simulink model "CAR_CONTROL_SYSTEM"  (R2024b)
settings: Solver=FixedStepAuto  StartTime=0.0  StopTime=inf  FixedStep=1e-3  RelTol=1e-3  EnableMultiTasking=on
model workspace (MAT data in the model file):
  SL_ROS_VariableLengthArrays_MaxSizes : object (value not decoded)
undefined symbols (not defined in the file or in its folder): angular, CIRCUIT, CLTF_DAMP, CLTF_FREQ, CLTF_GAIN, CONTROL, CONTROL_INI, DiscIntNeverNeededParam, dspblkCoreblockFVToolHelper, gcbh, INPUT, linear, MCP3201, MD25, MODEL, MODEL_INI, mpcstate, MPU60X0, MPU9250, MSG, NAV_MPC_CONTROL, OUTPUT, SAMPLING_TIME, SYSID_INPUT, VL6180X
libraries: raspberrypiCommlib x153, simulink x85, raspberrypiNetworklib x8, embedlinuxBasiclib x6, ctrlSharedLib x2, ros2lib x2, mpclib x1, vrlib x1, sldrtlib x1
(part 4 of 16)

== system CAR_CONTROL_SYSTEM/HARDWARE/SENSORS/RCRX iBUS ==
  BUS UPDATE : MATLAB Function  Priority=20  TreatAsAtomicUnit=on
  Data Store Read19 : DataStoreRead  DataStoreName=CONTROL  SampleTime=SAMPLING_TIME  IndexOptions=Index vector (dialog)  Indices=1  OutputSizes=1
  Data Store Write1 : DataStoreWrite  DataStoreName=CONTROL  IndexOptions=Index vector (dialog)  Indices=1  OutputSizes=1
  Display3 : Display
  MATLAB Function : MATLAB Function  TreatAsAtomicUnit=on
  Serial Read1 : raspberrypiCommlib/Serial Read  board=Pi 3 Model B  SCIModule_=/dev/ttyS0  Baudrate_=115200  Parity=None  StopBits_=1  HardwareFlowControl=None  ByteOrder=LittleEndian  DataLength=70  DataType=uint8  OutputStatus=on  SampleTime=SAMPLING_TIME  blockPlatform=RaspberryPi
  Terminator : Terminator
  wires:
  MATLAB Function/1(CH_RAW) -> BUS UPDATE/2(CH_RAW)
  BUS UPDATE/1(CONTROL) -> Data Store Write1/1
  Data Store Read19/1 -> BUS UPDATE/1(CONTROL_IN)
  Serial Read1/1 -> MATLAB Function/1(iBUS_DATA), Display3/1
  Serial Read1/2 -> Terminator/1

== system CAR_CONTROL_SYSTEM/HARDWARE/SENSORS/WALL RANGE SENSOR ==
  ANGLE AND DISTANCE COMPUTATION : Subsystem  TreatAsAtomicUnit=on
      settings: MinAlgLoopOccurrences=on
  Data Store Memory : DataStoreMemory  DataStoreName=REAR_DISTANCE  ReadBeforeWriteMsg=warning  WriteAfterWriteMsg=warning  WriteAfterReadMsg=warning  ShowAdditionalParam=off  OutDataTypeStr=double
  Data Store Memory1 : DataStoreMemory  DataStoreName=FRONT_DISTANCE  ReadBeforeWriteMsg=warning  WriteAfterWriteMsg=warning  WriteAfterReadMsg=warning  ShowAdditionalParam=off  OutDataTypeStr=double
  VL6180X_I2C_FRONT : Subsystem  TreatAsAtomicUnit=on
      settings: MinAlgLoopOccurrences=on  RTWSystemCode=Nonreusable function  FunctionWithSeparateData=on
  VL6180X_I2C_REAR : Subsystem  TreatAsAtomicUnit=on
      settings: MinAlgLoopOccurrences=on  RTWSystemCode=Nonreusable function  FunctionWithSeparateData=on

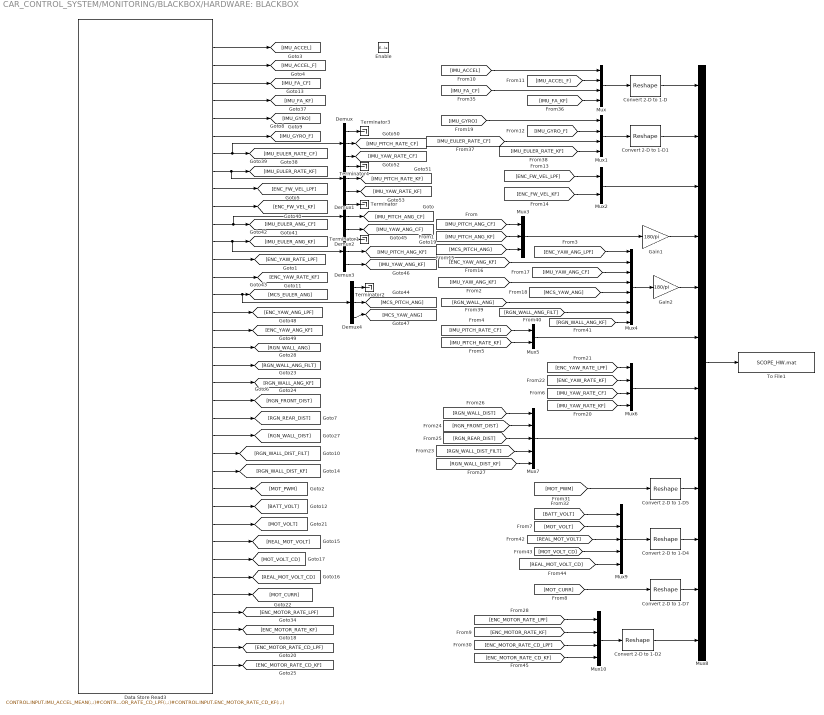
== system CAR_CONTROL_SYSTEM/MONITORING/BLACKBOX/HARDWARE: BLACKBOX ==
  Enable : EnablePort
  Convert 2-D to 1-D{,1..2,4..5,7} (6 alike) : Reshape
  Data Store Read3 : DataStoreRead  DataStoreName=CONTROL  SampleTime=SAMPLING_TIME  DataStoreElements=CONTROL.INPUT.IMU_ACCEL_MEAN(:,:)#CONTROL.INPUT.IMU_ACCEL_MEAN_FILT(:,:)#CONTROL.INPUT.IMU_FORWARD_ACCEL_CF#CONTROL.INPUT.IMU_FORWARD_ACCEL_KF#CONTROL.INPUT.IMU_GYRO_MEAN(:,:)#CONTROL.INPUT.IMU_GYRO_MEAN_FILT(:,:)#CONTROL.INPUT.IMU_EULER_RATE_CF(:,:)#CONTROL.INPUT.IMU_EULER_RATE_KF(:,:)#CONTROL.INPUT.ENC_FORWARD_VEL_LPF#CONTROL.INPUT.ENC_FORWARD_VEL_KF#CONTROL.INPUT.IMU_EULER_ANG_CF(:,:)#CONTROL.INPUT.IMU_EULER_ANG_KF(:,:)#CONTROL.INPUT.ENC_YAW_RATE_LPF#CONTROL.INPUT.ENC_YAW_RATE_KF#CONTROL.INPUT.MCS_EULER_ANG(:,:)#CONTROL.INPUT.ENC_YAW_ANG_LPF#CONTROL.INPUT.ENC_YAW_ANG_KF#CONTROL.INPUT.RANGE_WALL_ANG#CONTROL.INPUT.WALL_ANG_FILT#CONTROL.INPUT.WALL_ANG_KF#CONTROL.INPUT.RANGE_FRONT_DIST#CONTROL.INPUT.RANGE_REAR_DIST#CONTROL.INPUT.RANGE_WALL_DIST#CONTROL.INPUT.WALL_DIST_FILT#CONTROL.INPUT.WALL_DIST_KF#CONTROL.OUTPUT.MOTOR_PWM(:,:)#CONTROL.INPUT.BATTERY_VOLT#CONTROL.OUTPUT.MOTOR_VOLT(:,:)#CONTROL.OUTPUT.REAL_MOTOR_VOLT(:,:)#CONTROL.OUTPUT.MOTOR_VOLT_CD(:,:)#CONTROL.OUTPUT.REAL_MOTOR_VOLT_CD(:,:)#CONTROL.INPUT.MOTOR_CURRENT(:,:)#CONTROL.INPUT.ENC_MOTOR_RATE_LPF(:,:)#CONTROL.INPUT.ENC_MOTOR_RATE_KF(:,:)#CONTROL.INPUT.ENC_MOTOR_RATE_CD_LPF(:,:)#CONTROL.INPUT.ENC_MOTOR_RATE_CD_KF(:,:)  IndexOptions=Index vector (dialog)  Indices=1  OutputSizes=1
  Demux{,1..4} (5 alike) : Demux  Outputs=3
  Gain1 : Gain  Gain=180/pi
  Gain2 : Gain  Gain=180/pi
  Mux{,1,6,10} (4 alike) : Mux
  Mux2 : Mux  Inputs=2
  Mux3 : Mux  Inputs=3
  Mux4 : Mux  Inputs=8
  Mux5 : Mux  Inputs=2
  Mux7 : Mux  Inputs=5
  Mux8 : Mux  Inputs=12
  Mux9 : Mux  Inputs=5
  Terminator{,1..4} (5 alike) : Terminator
  To File1 : ToFile  Filename=SCOPE_HW.mat  MatrixName=SCOPE_HW  SampleTime=SAMPLING_TIME
  wires:
  [MOT_CURR] -> Convert 2-D to 1-D7/1
  Convert 2-D to 1-D/1 -> Mux8/1
  Convert 2-D to 1-D1/1 -> Mux8/2
  Mux2/1 -> Mux8/3
  [IMU_ACCEL] -> Mux/1
  Mux/1 -> Convert 2-D to 1-D/1
  [IMU_ACCEL_F] -> Mux/2
  [ENC_FW_VEL_LPF] -> Mux2/1
  [ENC_FW_VEL_KF] -> Mux2/2
  [IMU_PITCH_ANG_CF] -> Mux3/1
  [IMU_PITCH_ANG_KF] -> Mux3/2
  Mux3/1 -> Gain1/1
  Gain1/1 -> Mux8/4
  Mux4/1 -> Gain2/1
  Gain2/1 -> Mux8/5
  Mux5/1 -> Mux8/6
  [IMU_PITCH_RATE_CF] -> Mux5/1
  [IMU_PITCH_RATE_KF] -> Mux5/2
  Mux6/1 -> Mux8/7
  Mux7/1 -> Mux8/8
  [RGN_WALL_DIST] -> Mux7/1
  [RGN_FRONT_DIST] -> Mux7/2
  [RGN_REAR_DIST] -> Mux7/3
  Mux9/1 -> Convert 2-D to 1-D4/1
  [MOT_VOLT] -> Mux9/2
  [BATT_VOLT] -> Mux9/1
  [MOT_PWM] -> Convert 2-D to 1-D5/1
  Convert 2-D to 1-D5/1 -> Mux8/9
  Convert 2-D to 1-D4/1 -> Mux8/10
  Convert 2-D to 1-D7/1 -> Mux8/11
  Data Store Read3/1 -> [IMU_ACCEL]
  Data Store Read3/2 -> [IMU_ACCEL_F]
  [ENC_MOTOR_RATE_KF] -> Mux10/2
  Mux10/1 -> Convert 2-D to 1-D2/1
  [ENC_MOTOR_RATE_LPF] -> Mux10/1
  Data Store Read3/32 -> [MOT_CURR]
  Data Store Read3/33 -> [ENC_MOTOR_RATE_LPF]
  Data Store Read3/34 -> [ENC_MOTOR_RATE_KF]
  Data Store Read3/5 -> [IMU_GYRO]
  Data Store Read3/6 -> [IMU_GYRO_F]
  Data Store Read3/3 -> [IMU_FA_CF]
  Data Store Read3/4 -> [IMU_FA_KF]
  [IMU_FA_CF] -> Mux/3
  [IMU_FA_KF] -> Mux/4
  Data Store Read3/7 -> Demux/1, [IMU_EULER_RATE_CF]
  Data Store Read3/8 -> Demux1/1, [IMU_EULER_RATE_KF]
  Mux1/1 -> Convert 2-D to 1-D1/1
  [IMU_GYRO] -> Mux1/1
  [IMU_GYRO_F] -> Mux1/2
  [IMU_EULER_RATE_CF] -> Mux1/3
  [IMU_EULER_RATE_KF] -> Mux1/4
  Data Store Read3/9 -> [ENC_FW_VEL_LPF]
  Data Store Read3/10 -> [ENC_FW_VEL_KF]
  Data Store Read3/11 -> Demux2/1, [IMU_EULER_ANG_CF]
  Data Store Read3/12 -> Demux3/1, [IMU_EULER_ANG_KF]
  Demux2/2 -> [IMU_PITCH_ANG_CF]
  Demux3/2 -> [IMU_PITCH_ANG_KF]
  Demux4/2 -> [MCS_PITCH_ANG]
  [MCS_PITCH_ANG] -> Mux3/3
  Demux2/3 -> [IMU_YAW_ANG_CF]
  Demux3/3 -> [IMU_YAW_ANG_KF]
  Demux2/1 -> Terminator/1
  Demux3/1 -> Terminator1/1
  Demux4/3 -> [MCS_YAW_ANG]
  Demux4/1 -> Terminator2/1
  [ENC_YAW_ANG_LPF] -> Mux4/1
  [ENC_YAW_ANG_KF] -> Mux4/2
  [IMU_YAW_ANG_CF] -> Mux4/3
  [IMU_YAW_ANG_KF] -> Mux4/4
  [MCS_YAW_ANG] -> Mux4/5
  [RGN_WALL_ANG] -> Mux4/6
  [RGN_WALL_ANG_FILT] -> Mux4/7
  [RGN_WALL_ANG_KF] -> Mux4/8
  Demux/2 -> [IMU_PITCH_RATE_CF]
  Demux1/2 -> [IMU_PITCH_RATE_KF]
  Demux/1 -> Terminator3/1
  Demux1/1 -> Terminator4/1
  Demux/3 -> [IMU_YAW_RATE_CF]
  Demux1/3 -> [IMU_YAW_RATE_KF]
  Data Store Read3/14 -> [ENC_YAW_RATE_KF]
  Data Store Read3/15 -> Demux4/1, [MCS_EULER_ANG]
  Data Store Read3/16 -> [ENC_YAW_ANG_LPF]
  Data Store Read3/17 -> [ENC_YAW_ANG_KF]
  Data Store Read3/18 -> [RGN_WALL_ANG]
  Data Store Read3/19 -> [RGN_WALL_ANG_FILT]
  Data Store Read3/20 -> [RGN_WALL_ANG_KF]
  Data Store Read3/13 -> [ENC_YAW_RATE_LPF]
  Data Store Read3/21 -> [RGN_FRONT_DIST]
  Data Store Read3/22 -> [RGN_REAR_DIST]
  Data Store Read3/23 -> [RGN_WALL_DIST]
  Data Store Read3/24 -> [RGN_WALL_DIST_FILT]
  Data Store Read3/25 -> [RGN_WALL_DIST_KF]
  [RGN_WALL_DIST_FILT] -> Mux7/4
  [RGN_WALL_DIST_KF] -> Mux7/5
  Data Store Read3/26 -> [MOT_PWM]
  Data Store Read3/27 -> [BATT_VOLT]
  Data Store Read3/28 -> [MOT_VOLT]
  Data Store Read3/29 -> [REAL_MOT_VOLT]
  Data Store Read3/31 -> [REAL_MOT_VOLT_CD]
  Data Store Read3/30 -> [MOT_VOLT_CD]
  [REAL_MOT_VOLT_CD] -> Mux9/5
  [REAL_MOT_VOLT] -> Mux9/3
  [MOT_VOLT_CD] -> Mux9/4
  Data Store Read3/35 -> [ENC_MOTOR_RATE_CD_LPF]
  Data Store Read3/36 -> [ENC_MOTOR_RATE_CD_KF]
  [ENC_MOTOR_RATE_CD_LPF] -> Mux10/3
  [ENC_MOTOR_RATE_CD_KF] -> Mux10/4
  Convert 2-D to 1-D2/1 -> Mux8/12
  [IMU_YAW_RATE_CF] -> Mux6/3
  [IMU_YAW_RATE_KF] -> Mux6/4
  [ENC_YAW_RATE_LPF] -> Mux6/1
  [ENC_YAW_RATE_KF] -> Mux6/2
  Mux8/1 -> To File1/1

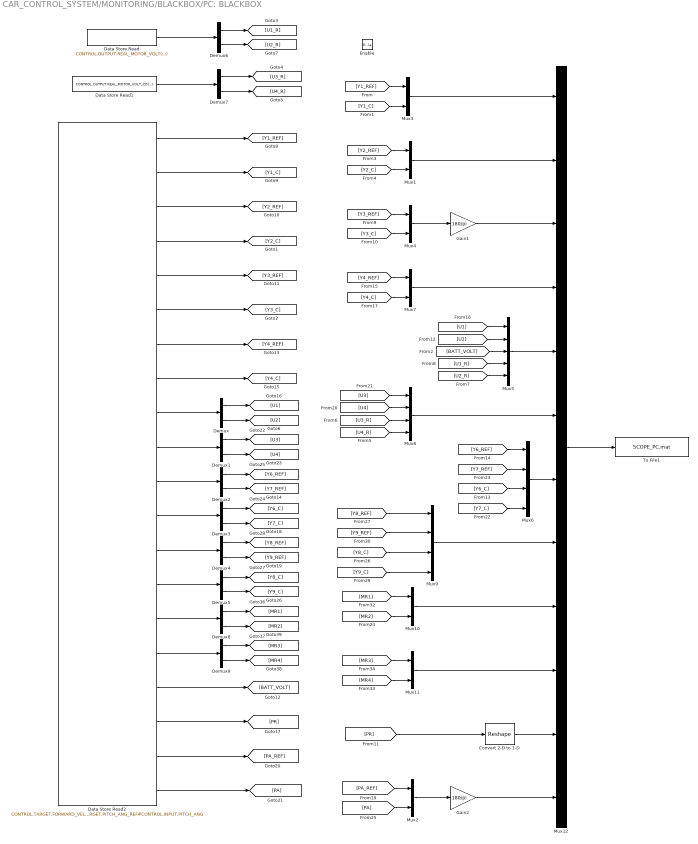
== system CAR_CONTROL_SYSTEM/MONITORING/BLACKBOX/PC: BLACKBOX ==
  Enable : EnablePort
  Convert 2-D to 1-D : Reshape
  Data Store Read : DataStoreRead  DataStoreName=CONTROL  DataStoreElements=CONTROL.OUTPUT.REAL_MOTOR_VOLT(:,:)  IndexOptions=Index vector (dialog)  Indices=1  OutputSizes=1
  Data Store Read1 : DataStoreRead  DataStoreName=CONTROL  DataStoreElements=CONTROL.OUTPUT.REAL_MOTOR_VOLT_CD(:,:)  IndexOptions=Index vector (dialog)  Indices=1  OutputSizes=1
  Data Store Read2 : DataStoreRead  DataStoreName=CONTROL  SampleTime=SAMPLING_TIME  DataStoreElements=CONTROL.TARGET.FORWARD_VEL_REF#CONTROL.INPUT.FORWARD_VEL#CONTROL.TARGET.YAW_RATE_REF#CONTROL.INPUT.YAW_RATE#CONTROL.TARGET.YAW_ANG_REF#CONTROL.INPUT.YAW_ANG#CONTROL.TARGET.WALL_DIST_REF#CONTROL.INPUT.WALL_DIST#CONTROL.OUTPUT.MOTOR_VOLT(:,:)#CONTROL.OUTPUT.MOTOR_VOLT_CD(:,:)#CONTROL.TARGET.POS_XY_REF(:,:)#CONTROL.INPUT.EARTH_POS(1:2,1)#CONTROL.TARGET.VEL_XY_REF(:,:)#CONTROL.INPUT.EARTH_VEL(1:2,1)#CONTROL.INPUT.MOTOR_RATE(:,:)#CONTROL.INPUT.MOTOR_RATE_CD(:,:)#CONTROL.INPUT.BATTERY_VOLT#CONTROL.INPUT.PITCH_RATE#CONTROL.TARGET.PITCH_ANG_REF#CONTROL.INPUT.PITCH_ANG  IndexOptions=Index vector (dialog)  Indices=1  OutputSizes=1
  Demux{,1..9} (10 alike) : Demux  Outputs=2
  Gain1 : Gain  Gain=180/pi
  Gain2 : Gain  Gain=180/pi
  Mux{1..4,7,10..11} (7 alike) : Mux  Inputs=2
  Mux12 : Mux  Inputs=12
  Mux5 : Mux  Inputs=5
  Mux6 : Mux
  Mux8 : Mux
  Mux9 : Mux
  To File1 : ToFile  Filename=SCOPE_PC.mat  MatrixName=SCOPE_PC  SampleTime=SAMPLING_TIME
  wires:
  Gain2/1 -> Mux12/12
  Data Store Read2/17 -> [BATT_VOLT]
  [PR] -> Convert 2-D to 1-D/1
  Data Store Read2/7 -> [Y4_REF]
  Data Store Read2/5 -> [Y3_REF]
  [Y4_C] -> Mux7/2
  Data Store Read2/1 -> [Y1_REF]
  Data Store Read2/14 -> Demux5/1
  Demux8/1 -> [MR1]
  Data Store Read2/4 -> [Y2_C]
  Data Store Read2/2 -> [Y1_C]
  [MR1] -> Mux10/1
  Demux7/2 -> [U4_R]
  [Y9_C] -> Mux9/4
  Demux5/2 -> [Y9_C]
  [PA] -> Mux2/2
  [U4] -> Mux8/2
  [MR3] -> Mux11/1
  Demux1/2 -> [U4]
  Data Store Read2/16 -> Demux9/1
  Demux4/2 -> [Y9_REF]
  Data Store Read2/8 -> [Y4_C]
  [Y1_C] -> Mux3/2
  [Y1_REF] -> Mux3/1
  [U2] -> Mux5/2
  Demux/2 -> [U2]
  Mux1/1 -> Mux12/2
  Demux7/1 -> [U3_R]
  [Y9_REF] -> Mux9/2
  Data Store Read2/18 -> [PR]
  Demux6/1 -> [U1_R]
  Mux9/1 -> Mux12/8
  [Y7_C] -> Mux6/4
  [Y2_C] -> Mux1/2
  Mux6/1 -> Mux12/7
  Mux12/1 -> To File1/1
  Demux2/2 -> [Y7_REF]
  Data Store Read2/12 -> Demux3/1
  Data Store Read2/9 -> Demux/1
  [Y3_C] -> Mux4/2
  [Y2_REF] -> Mux1/1
  Data Store Read2/15 -> Demux8/1
  Mux3/1 -> Mux12/1
  [MR4] -> Mux11/2
  Mux10/1 -> Mux12/9
  [Y6_C] -> Mux6/3
  Data Store Read2/10 -> Demux1/1
  Mux4/1 -> Gain1/1
  Demux1/1 -> [U3]
  [Y8_REF] -> Mux9/1
  Data Store Read/1 -> Demux6/1
  Demux4/1 -> [Y8_REF]
  Demux3/2 -> [Y7_C]
  Demux2/1 -> [Y6_REF]
  Demux3/1 -> [Y6_C]
  [Y3_REF] -> Mux4/1
  [PA_REF] -> Mux2/1
  [Y6_REF] -> Mux6/1
  Data Store Read2/11 -> Demux2/1
  [U3_R] -> Mux8/3
  Demux6/2 -> [U2_R]
  Mux5/1 -> Mux12/5
  Mux8/1 -> Mux12/6
  Demux8/2 -> [MR2]
  Gain1/1 -> Mux12/3
  [Y7_REF] -> Mux6/2
  Mux7/1 -> Mux12/4
  Data Store Read2/13 -> Demux4/1
  Data Store Read2/19 -> [PA_REF]
  Demux/1 -> [U1]
  [U4_R] -> Mux8/4
  [U1_R] -> Mux5/4
  Mux2/1 -> Gain2/1
  Convert 2-D to 1-D/1 -> Mux12/11
  Demux5/1 -> [Y8_C]
  [Y4_REF] -> Mux7/1
  Demux9/2 -> [MR4]
  Data Store Read2/6 -> [Y3_C]
  Mux11/1 -> Mux12/10
  [U2_R] -> Mux5/5
  Data Store Read1/1 -> Demux7/1
  Data Store Read2/3 -> [Y2_REF]
  [U1] -> Mux5/1
  Demux9/1 -> [MR3]
  [Y8_C] -> Mux9/3
  Data Store Read2/20 -> [PA]
  [U3] -> Mux8/1
  [BATT_VOLT] -> Mux5/3
  [MR2] -> Mux10/2

== system CAR_CONTROL_SYSTEM/MONITORING/COMMUNICATIONS/MSG_RX ==
  Enable : EnablePort
  Data Store Read : DataStoreRead  DataStoreName=MSG  SampleTime=CONTROL_INI.PARAM.COMM_SAMPLING_TIME  IndexOptions=Index vector (dialog)  Indices=1  OutputSizes=1
  Data Store Read2 : DataStoreRead  DataStoreName=CONTROL  SampleTime=CONTROL_INI.PARAM.COMM_SAMPLING_TIME  IndexOptions=Index vector (dialog)  Indices=1  OutputSizes=1
  Data Store Write1 : DataStoreWrite  DataStoreName=MSG  SampleTime=CONTROL_INI.PARAM.COMM_SAMPLING_TIME  IndexOptions=Index vector (dialog)  Indices=1  OutputSizes=1
  Data Store Write2 : DataStoreWrite  DataStoreName=CONTROL  SampleTime=CONTROL_INI.PARAM.COMM_SAMPLING_TIME  IndexOptions=Index vector (dialog)  Indices=1  OutputSizes=1
  MSG DECODER : MATLAB Function  Priority=20  TreatAsAtomicUnit=on
  wires:
  Data Store Read2/1 -> MSG DECODER/2(CONTROL_IN)
  MSG DECODER/1(MSG) -> Data Store Write1/1
  Data Store Read/1 -> MSG DECODER/1(MSG_IN)
  MSG DECODER/2(CONTROL) -> Data Store Write2/1

== system CAR_CONTROL_SYSTEM/MONITORING/COMMUNICATIONS/MSG_TX  ==
  Enable : EnablePort
  Data Store Read : DataStoreRead  DataStoreName=MSG  SampleTime=CONTROL_INI.PARAM.COMM_SAMPLING_TIME  IndexOptions=Index vector (dialog)  Indices=1  OutputSizes=1
  Data Store Read6 : DataStoreRead  DataStoreName=CONTROL  SampleTime=CONTROL_INI.PARAM.COMM_SAMPLING_TIME  IndexOptions=Index vector (dialog)  Indices=1  OutputSizes=1
  Data Store Write1 : DataStoreWrite  DataStoreName=MSG  SampleTime=CONTROL_INI.PARAM.COMM_SAMPLING_TIME  IndexOptions=Index vector (dialog)  Indices=1  OutputSizes=1
  MSG CODER : MATLAB Function  Priority=20  TreatAsAtomicUnit=on
  wires:
  Data Store Read/1 -> MSG CODER/1(MSG_IN)
  MSG CODER/1(MSG) -> Data Store Write1/1
  Data Store Read6/1 -> MSG CODER/2(CONTROL)

== system CAR_CONTROL_SYSTEM/MONITORING/ROS_COM/DYNAMICS PUBLISHERS ==
  Blank Message : ros2lib/Blank Message  messageClass=Message  entityType=geometry_msgs/Twist  messageType=geometry_msgs/Twist  SampleTime=-1
  Bus Assignment : BusAssignment  AssignedSignals=linear.x,linear.y,linear.z,angular.x,angular.y,angular.z
  Constant{,1..3} (4 alike) : Constant  Value=0  SampleTime=SAMPLING_TIME
  Data Store Read : DataStoreRead  DataStoreName=MODEL  SampleTime=SAMPLING_TIME  DataStoreElements=MODEL.OUTPUT.FORWARD_VEL#MODEL.OUTPUT.YAW_RATE  IndexOptions=Index vector (dialog)  Indices=1  OutputSizes=1
  Data Type Conversion4 : DataTypeConversion  SaturateOnIntegerOverflow=off  RndMeth=Floor
  Data Type Conversion9 : DataTypeConversion  SaturateOnIntegerOverflow=off  RndMeth=Floor
  Gain : Gain  Gain=-1
  POSE SCOPE : Scope  NumInputPorts=2
  Publish : ros2lib/Publish  topicSource=Specify your own  topic=/cmd_vel  messageType=geometry_msgs/Twist  QOSHistory=Keep last  QOSDepth=1  QOSReliability=Reliable  QOSDurability=Volatile  QOSDeadline=Inf  QOSLifespan=Inf  QOSLiveliness=Automatic  QOSLeaseDuration=Inf  QOSAvoidROSNamespaceConventions=off
  wires:
  Constant1/1 -> Bus Assignment/4
  [CAR_YR] -> Gain/1
  Constant2/1 -> Bus Assignment/5
  [CAR_FV] -> Data Type Conversion4/1
  Data Store Read/2 -> [CAR_YR]
  Bus Assignment/1 -> Publish/1
  [CAR_FV] -> POSE SCOPE/1  "FV"
  Constant3/1 -> Bus Assignment/6
  Data Type Conversion4/1 -> Bus Assignment/2
  Data Type Conversion9/1 -> Bus Assignment/7
  [CAR_YR] -> POSE SCOPE/2  "YR"
  Blank Message/1 -> Bus Assignment/1
  Data Store Read/1 -> [CAR_FV]
  Constant/1 -> Bus Assignment/3
  Gain/1 -> Data Type Conversion9/1

== system CAR_CONTROL_SYSTEM/MONITORING/SIMULATION: SCOPES/Second-order LPF 1 ==
  In : Inport
  Discrete Transfer Fcn : DiscreteTransferFcn  Numerator=Fd.num{1}  Denominator=Fd.den{1}  SampleTime=ts
  Out : Outport  VectorParamsAs1DForOutWhenUnconnected=off
  wires:
  In/1 -> Discrete Transfer Fcn/1
  Discrete Transfer Fcn/1 -> Out/1

== system CAR_CONTROL_SYSTEM/MONITORING/SIMULATION: SCOPES/Second-order LPF 2 ==
  In : Inport
  Discrete Transfer Fcn : DiscreteTransferFcn  Numerator=Fd.num{1}  Denominator=Fd.den{1}  SampleTime=ts
  Out : Outport  VectorParamsAs1DForOutWhenUnconnected=off
  wires:
  In/1 -> Discrete Transfer Fcn/1
  Discrete Transfer Fcn/1 -> Out/1

== system CAR_CONTROL_SYSTEM/MONITORING/SIMULATION: SCOPES/Second-order LPF 3 ==
  In : Inport
  Discrete Transfer Fcn : DiscreteTransferFcn  Numerator=Fd.num{1}  Denominator=Fd.den{1}  SampleTime=ts
  Out : Outport  VectorParamsAs1DForOutWhenUnconnected=off
  wires:
  In/1 -> Discrete Transfer Fcn/1
  Discrete Transfer Fcn/1 -> Out/1

== system CAR_CONTROL_SYSTEM/MONITORING/SIMULATION: SCOPES/Second-order LPF 4 ==
  In : Inport
  Discrete Transfer Fcn : DiscreteTransferFcn  Numerator=Fd.num{1}  Denominator=Fd.den{1}  SampleTime=ts
  Out : Outport  VectorParamsAs1DForOutWhenUnconnected=off
  wires:
  In/1 -> Discrete Transfer Fcn/1
  Discrete Transfer Fcn/1 -> Out/1

== system CAR_CONTROL_SYSTEM/MONITORING/SIMULATION: SCOPES/Second-order LPF 5 ==
  In : Inport
  Discrete Transfer Fcn : DiscreteTransferFcn  Numerator=Fd.num{1}  Denominator=Fd.den{1}  SampleTime=ts
  Out : Outport  VectorParamsAs1DForOutWhenUnconnected=off
  wires:
  In/1 -> Discrete Transfer Fcn/1
  Discrete Transfer Fcn/1 -> Out/1

== system CAR_CONTROL_SYSTEM/SIMULATION/RC TRANSMITTER /SWB ==
  UP : Inport
  DOWN : Inport  Port=2
  Constant1 : Constant  Value=1500  SampleTime=-1
  Gain : Gain  Gain=-500
  Gain5 : Gain  Gain=500
  Sum : Sum  Inputs=3
  SWITCH : Outport
  wires:
  Constant1/1 -> Sum/2
  Sum/1 -> SWITCH/1
  UP/1 -> Gain/1
  Gain5/1 -> Sum/3
  Gain/1 -> Sum/1
  DOWN/1 -> Gain5/1

== system CAR_CONTROL_SYSTEM/SIMULATION/RC TRANSMITTER /SWC ==
  UP : Inport
  DOWN : Inport  Port=2
  Constant1 : Constant  Value=1500  SampleTime=-1
  Gain : Gain  Gain=-500
  Gain5 : Gain  Gain=500
  Sum : Sum  Inputs=3
  SWITCH : Outport
  wires:
  DOWN/1 -> Gain5/1
  Gain/1 -> Sum/1
  Gain5/1 -> Sum/3
  UP/1 -> Gain/1
  Sum/1 -> SWITCH/1
  Constant1/1 -> Sum/2

== system CAR_CONTROL_SYSTEM/SIMULATION/READ IMU/ LPF 3 ==
  IN : Inport
  ALFA : Inport  Port=2  SampleTime=MPU60X0.SAMPLING_TIME
  Bias : Bias  Bias=single(1)  SaturateOnIntegerOverflow=off
  Gain : Gain  Gain=-1
  Product : Product
  Product2 : Product
  Sum : Sum  Inputs=|++
  Unit Delay : UnitDelay  SampleTime=-1  HasFrameUpgradeWarning=on
  OUT : Outport  VectorParamsAs1DForOutWhenUnconnected=off
  wires:
  IN/1 -> Product2/1
  Bias/1 -> Product2/2
  Product2/1 -> Sum/1
  Gain/1 -> Bias/1
  ALFA/1 -> Product/2, Gain/1
  Sum/1 -> OUT/1, Unit Delay/1
  Product/1 -> Sum/2
  Unit Delay/1 -> Product/1

== system CAR_CONTROL_SYSTEM/SIMULATION/READ IMU/ LPF 4 ==
  IN : Inport
  ALFA : Inport  Port=2  SampleTime=MPU60X0.SAMPLING_TIME
  Bias : Bias  Bias=single(1)  SaturateOnIntegerOverflow=off
  Gain : Gain  Gain=-1
  Product : Product
  Product2 : Product
  Sum : Sum  Inputs=|++
  Unit Delay : UnitDelay  SampleTime=-1  HasFrameUpgradeWarning=on
  OUT : Outport  VectorParamsAs1DForOutWhenUnconnected=off
  wires:
  IN/1 -> Product2/1
  Bias/1 -> Product2/2
  Product2/1 -> Sum/1
  Gain/1 -> Bias/1
  ALFA/1 -> Product/2, Gain/1
  Sum/1 -> OUT/1, Unit Delay/1
  Product/1 -> Sum/2
  Unit Delay/1 -> Product/1

== system CAR_CONTROL_SYSTEM/SIMULATION/READ IMU/FILTER POLE ==
  Constant : Constant  Value=MPU60X0.SAMPLING_TIME  OutDataTypeStr=single  SampleTime=MPU60X0.SAMPLING_TIME
  Data Store Read4 : DataStoreRead  DataStoreName=CONTROL  SampleTime=MPU60X0.SAMPLING_TIME  DataStoreElements=CONTROL.PARAM.IMU_FILT_FREQ  IndexOptions=Index vector (dialog)  Indices=1  OutputSizes=1
  Gain : Gain  Gain=-2*pi
  Math Function : Math  SignedPower=on
  Product1 : Product
  ALFA : Outport  VectorParamsAs1DForOutWhenUnconnected=off
  wires:
  Data Store Read4/1 -> Gain/1
  Product1/1 -> Math Function/1
  Constant/1 -> Product1/1
  Math Function/1 -> ALFA/1
  Gain/1 -> Product1/2

== system CAR_CONTROL_SYSTEM/SIMULATION/READ IMU/LPF 1 ==
  IN : Inport
  ALFA : Inport  Port=2  SampleTime=MPU60X0.SAMPLING_TIME
  Bias : Bias  Bias=single(1)  SaturateOnIntegerOverflow=off
  Gain : Gain  Gain=-1
  Product : Product
  Product2 : Product
  Sum : Sum  Inputs=|++
  Unit Delay : UnitDelay  InitialCondition=[CONTROL_INI.PARAM.GRAVITY*CONTROL_INI.STATE.VEHICLE_MODE ; 0 ; -CONTROL_INI.PARAM.GRAVITY*(1-CONTROL_INI.STATE.VEHICLE_MODE)]  SampleTime=-1  HasFrameUpgradeWarning=on
  OUT : Outport  VectorParamsAs1DForOutWhenUnconnected=off
  wires:
  Unit Delay/1 -> Product/1
  Product/1 -> Sum/2
  Sum/1 -> Unit Delay/1, OUT/1
  ALFA/1 -> Gain/1, Product/2
  Gain/1 -> Bias/1
  Product2/1 -> Sum/1
  Bias/1 -> Product2/2
  IN/1 -> Product2/1

== system CAR_CONTROL_SYSTEM/SIMULATION/READ IMU/LPF 2 2 ==
  IN : Inport
  ALFA : Inport  Port=2  SampleTime=MPU60X0.SAMPLING_TIME
  Bias : Bias  Bias=single(1)  SaturateOnIntegerOverflow=off
  Gain : Gain  Gain=-1
  Product : Product
  Product2 : Product
  Sum : Sum  Inputs=|++
  Unit Delay : UnitDelay  InitialCondition=[CONTROL_INI.PARAM.GRAVITY*CONTROL_INI.STATE.VEHICLE_MODE ; 0 ; -CONTROL_INI.PARAM.GRAVITY*(1-CONTROL_INI.STATE.VEHICLE_MODE)]  SampleTime=-1  HasFrameUpgradeWarning=on
  OUT : Outport  VectorParamsAs1DForOutWhenUnconnected=off
  wires:
  Unit Delay/1 -> Product/1
  Product/1 -> Sum/2
  Sum/1 -> Unit Delay/1, OUT/1
  ALFA/1 -> Gain/1, Product/2
  Gain/1 -> Bias/1
  Product2/1 -> Sum/1
  Bias/1 -> Product2/2
  IN/1 -> Product2/1

== system CAR_CONTROL_SYSTEM/GAZEBO SIMULATION/TCP_BRIDGE/TCP//IP PC/MSG_RX ==
  Bus Assignment : BusAssignment  AssignedSignals=RX_BUFFER
  Data Store Read : DataStoreRead  DataStoreName=MSG  IndexOptions=Index vector (dialog)  Indices=1  OutputSizes=1
  Data Store Write1 : DataStoreWrite  DataStoreName=MSG  IndexOptions=Index vector (dialog)  Indices=1  OutputSizes=1
  TCP/IP Receive : raspberrypiNetworklib/TCP//IP Receive  Mode_=Server  LocalServerPort_=27001  RemoteAddr_=127.0.0.1  RemoteServerPort_=25000  DataType_=uint8  DataSize_=1400  SampleTime_=CONTROL_INI.PARAM.COMM_SAMPLING_TIME  SimulateUsing=Code generation  ClientPortBindingSelection_=off  ClientPortToBind_=35000  BlockingMode_=off  BlockTimeout_=0.1  BlockPlatform=RASPBERRYPI
  Terminator1 : Terminator
  wires:
  TCP/IP Receive/1 -> Bus Assignment/2
  Data Store Read/1 -> Bus Assignment/1
  Bus Assignment/1 -> Data Store Write1/1
  TCP/IP Receive/2 -> Terminator1/1

== system CAR_CONTROL_SYSTEM/GAZEBO SIMULATION/TCP_BRIDGE/TCP//IP PC/MSG_TX ==
  Enable : EnablePort
  Data Store Read1 : DataStoreRead  DataStoreName=MSG  SampleTime=CONTROL_INI.PARAM.COMM_SAMPLING_TIME  DataStoreElements=MSG.TX_BUFFER(:,1)  IndexOptions=Index vector (dialog)  Indices=1  OutputSizes=1
  TCP/IP Send : raspberrypiNetworklib/TCP//IP Send  Mode_=Server  LocalServerPort_=27000  RemoteAddr_=127.0.0.1  RemoteServerPort_=25000  SimulateUsing=Code generation  ClientPortBindingSelection_=off  ClientPortToBind_=35000  BlockingMode_=off  BlockTimeout_=0.1  BlockPlatform=RASPBERRYPI
  wires:
  Data Store Read1/1 -> TCP/IP Send/1

== system CAR_CONTROL_SYSTEM/GAZEBO SIMULATION/TCP_BRIDGE/TCP//IP SIM HW/Subsystem ==
  IMU : Inport
  " LPF 3" : Subsystem
  " LPF 4" : Subsystem
  Constant2 : Constant  Value=MPU60X0.ACCEL_CALIB  SampleTime=MPU60X0.SAMPLING_TIME
  Constant3 : Constant  Value=CONTROL_INI.PARAM.GRAVITY  SampleTime=MPU60X0.SAMPLING_TIME
  Constant4 : Constant  Value=MPU60X0.ALFA_CALIB  SampleTime=MPU60X0.SAMPLING_TIME
  Data Store Memory1 : DataStoreMemory  Priority=10  DataStoreName=MPU60X0_PITCH_OFFS  ReadBeforeWriteMsg=warning  WriteAfterWriteMsg=warning  WriteAfterReadMsg=warning  ShowAdditionalParam=off  OutDataTypeStr=double
  Data Store Memory5 : DataStoreMemory  Priority=10  DataStoreName=MPU60X0_ACCEL_OFFS  ReadBeforeWriteMsg=warning  WriteAfterWriteMsg=warning  WriteAfterReadMsg=warning  InitialValue=zeros(3,1)  ShowAdditionalParam=off  OutDataTypeStr=double
  Data Store Memory6 : DataStoreMemory  Priority=10  DataStoreName=MPU60X0_GYRO_OFFS  ReadBeforeWriteMsg=warning  WriteAfterWriteMsg=warning  WriteAfterReadMsg=warning  InitialValue=zeros(3,1)  ShowAdditionalParam=off  OutDataTypeStr=double
  Data Store Read : DataStoreRead  DataStoreName=CONTROL  SampleTime=MPU60X0.SAMPLING_TIME  DataStoreElements=CONTROL.STATE.VEHICLE_MODE  IndexOptions=Index vector (dialog)  Indices=1  OutputSizes=1
  Data Store Read1 : DataStoreRead  DataStoreName=MPU60X0_PITCH_OFFS  SampleTime=MPU60X0.SAMPLING_TIME  IndexOptions=Index vector (dialog)  Indices=1  OutputSizes=1
  Data Store Read6 : DataStoreRead  DataStoreName=MPU60X0_ACCEL_OFFS  SampleTime=MPU60X0.SAMPLING_TIME  IndexOptions=Index vector (dialog)  Indices=1  OutputSizes=1
  Data Store Read8 : DataStoreRead  DataStoreName=MPU60X0_GYRO_OFFS  SampleTime=MPU60X0.SAMPLING_TIME  IndexOptions=Index vector (dialog)  Indices=1  OutputSizes=1
  Data Store Read9 : DataStoreRead  DataStoreName=CONTROL  SampleTime=MPU60X0.SAMPLING_TIME  IndexOptions=Index vector (dialog)  Indices=1  OutputSizes=1
  Data Store Write3 : DataStoreWrite  DataStoreName=MPU60X0_ACCEL_OFFS  IndexOptions=Index vector (dialog)  Indices=1  OutputSizes=1
  Data Store Write4 : DataStoreWrite  DataStoreName=MPU60X0_GYRO_OFFS  IndexOptions=Index vector (dialog)  Indices=1  OutputSizes=1
  Data Store Write5 : DataStoreWrite  DataStoreName=CONTROL  IndexOptions=Index vector (dialog)  Indices=1  OutputSizes=1
  Demux : Demux  Outputs=2
  FILTER POLE : Subsystem
  GRAVITY ROTATION : MATLAB Function  TreatAsAtomicUnit=on
  IMU CALIBRATION : MATLAB Function  Priority=30  TreatAsAtomicUnit=on
  LPF 1 : Subsystem
  "LPF 2 " : Subsystem
  MEAN FILTER : DiscreteFilter  LoadFcn=dspblkCoreblockFVToolHelper(gcbh,'load');  Numerator=1/floor(SAMPLING_TIME*1000)*ones(1,floor(SAMPLING_TIME*1000))  Denominator=[1 zeros(1,floor(SAMPLING_TIME*1000)-1)]
      settings: CopyFcn=dspblkCoreblockFVToolHelper(gcbh,'copy');  DeleteFcn=dspblkCoreblockFVToolHelper(gcbh,'close');  ModelCloseFcn=dspblkCoreblockFVToolHelper(gcbh,'close');  PreSaveFcn=dspblkCoreblockFVToolHelper(gcbh,'presave');  PostSaveFcn=dspblkCoreblockFVToolHelper(gcbh,'postsave');  CloseFcn=dspblkCoreblockFVToolHelper(gcbh,'close');
  "MEAN FILTER " : DiscreteFilter  Numerator=1/floor(SAMPLING_TIME*1000)*ones(1,floor(SAMPLING_TIME*1000))  Denominator=[1 zeros(1,floor(SAMPLING_TIME*1000)-1)]
  Scope : Scope  NumInputPorts=2
  wires:
  LPF 1/1(OUT) -> IMU CALIBRATION/3(ACCEL_FILT)
  IMU CALIBRATION/2(ACCEL_OFFS_OUT) -> Data Store Write3/1
  Data Store Read1/1 -> GRAVITY ROTATION/1(PITCH_OFFSET)
  GRAVITY ROTATION/1(GRAVITY_VECTOR) -> IMU CALIBRATION/14(GRAVITY_VECTOR)
  IMU CALIBRATION/1(CONTROL) -> Data Store Write5/1
  Data Store Read6/1 -> IMU CALIBRATION/12(ACCEL_OFFS_IN)
  " LPF 3"/1(OUT) -> IMU CALIBRATION/7(GYRO_FILT)
  Constant3/1 -> GRAVITY ROTATION/2(GRAVITY)
  FILTER POLE/1(ALFA) -> " LPF 4"/2(ALFA), " LPF 3"/2(ALFA), LPF 1/2(ALFA), "LPF 2 "/2(ALFA)
  "LPF 2 "/1(OUT) -> IMU CALIBRATION/5(ACCEL_MEAN_FILT)
  Data Store Read/1 -> GRAVITY ROTATION/3(VEHICLE_MODE)
  Data Store Read8/1 -> IMU CALIBRATION/13(GYRO_OFFS_IN)
  Demux/2 -> "MEAN FILTER "/1, IMU CALIBRATION/6(GYRO), " LPF 3"/1(IN), Scope/2
  "MEAN FILTER "/1 -> IMU CALIBRATION/8(GYRO_MEAN), " LPF 4"/1(IN)
  IMU CALIBRATION/3(GYRO_OFFS_OUT) -> Data Store Write4/1
  Data Store Read9/1 -> IMU CALIBRATION/1(CONTROL_IN)
  Demux/1 -> Scope/1, IMU CALIBRATION/2(ACCEL), LPF 1/1(IN), MEAN FILTER/1
  MEAN FILTER/1 -> "LPF 2 "/1(IN), IMU CALIBRATION/4(ACCEL_MEAN)
  " LPF 4"/1(OUT) -> IMU CALIBRATION/9(GYRO_MEAN_FILT)
  Constant4/1 -> IMU CALIBRATION/11(ALFA_CALIB)
  Constant2/1 -> IMU CALIBRATION/10(ACCEL_CALIB)
  IMU/1 -> Demux/1

== system CAR_CONTROL_SYSTEM/HARDWARE/ACTUATORS/MD25_I2C/MD25 INITIALIZATION ==
  Enable : EnablePort
  Compare To Zero{,1..4} (5 alike) : simulink/Logic and Bit Operations/Compare To Zero  relop===  OutDataTypeStr=boolean
  Constant1 : Constant  Value=MD25.MODE_BYTE  OutDataTypeStr=uint8  SampleTime=SAMPLING_TIME
  Constant10 : Constant  Value=hex2dec('32')  OutDataTypeStr=uint8  SampleTime=SAMPLING_TIME
  Constant2 : Constant  Value=hex2dec('10')  OutDataTypeStr=uint8  SampleTime=SAMPLING_TIME
  Constant3 : Constant  Value=MD25.MODE_BYTE  OutDataTypeStr=uint8  SampleTime=SAMPLING_TIME
  Constant6 : Constant  Value=hex2dec('20')  OutDataTypeStr=uint8  SampleTime=SAMPLING_TIME
  Constant9 : Constant  Value=hex2dec('30')  OutDataTypeStr=uint8  SampleTime=SAMPLING_TIME
  Data Store Write2 : DataStoreWrite  DataStoreName=MD25_INIT  IndexOptions=Index vector (dialog)  Indices=1  OutputSizes=1
  Logical Operator : Logic  Priority=100  Inputs=6  AllPortsSameDT=off  OutDataTypeStr=boolean
  MD25.ACCEL_RATE : raspberrypiCommlib/I2C Controller Write  Priority=30  BoardProperty=Pi 3 Model B+  I2CModule=1  Mode=Master  SlaveAddress=MD25.ADDRESS  SlaveByteOrder=BigEndian  Direction=Transmitter  RegisterAddressMode=on  RegisterAddress=MD25.ACCEL_RATE  SlaveDataType=uint8  DataLength=1  NoAck=off  RepeatedStart=off  OutputStatus=on
  MD25.COMMAND 1 : raspberrypiCommlib/I2C Controller Write  Priority=10  BoardProperty=Pi 3 Model B+  I2CModule=1  Mode=Master  SlaveAddress=MD25.ADDRESS  SlaveByteOrder=BigEndian  Direction=Transmitter  RegisterAddressMode=on  RegisterAddress=MD25.COMMAND  SlaveDataType=uint8  DataLength=1  NoAck=off  RepeatedStart=off  OutputStatus=on
  MD25.COMMAND 2 : raspberrypiCommlib/I2C Controller Write  Priority=20  BoardProperty=Pi 3 Model B+  I2CModule=1  Mode=Master  SlaveAddress=MD25.ADDRESS  SlaveByteOrder=BigEndian  Direction=Transmitter  RegisterAddressMode=on  RegisterAddress=MD25.COMMAND  SlaveDataType=uint8  DataLength=1  NoAck=off  RepeatedStart=off  OutputStatus=on
  MD25.COMMAND 3 : raspberrypiCommlib/I2C Controller Write  Priority=30  BoardProperty=Pi 3 Model B+  I2CModule=1  Mode=Master  SlaveAddress=MD25.ADDRESS  SlaveByteOrder=BigEndian  Direction=Transmitter  RegisterAddressMode=on  RegisterAddress=MD25.COMMAND  SlaveDataType=uint8  DataLength=1  NoAck=off  RepeatedStart=off  OutputStatus=on
  MD25.MODE : raspberrypiCommlib/I2C Controller Write  Priority=0  BoardProperty=Pi 3 Model B+  I2CModule=1  Mode=Master  SlaveAddress=MD25.ADDRESS  SlaveByteOrder=BigEndian  Direction=Transmitter  RegisterAddressMode=on  RegisterAddress=MD25.MODE  SlaveDataType=uint8  DataLength=1  NoAck=off  RepeatedStart=off  OutputStatus=on
  MD25.MODE READ : raspberrypiCommlib/I2C Controller Read  Priority=40  BoardProperty=Pi 3 Model B+  I2CModule=1  Mode=Master  SlaveAddress=MD25.ADDRESS  SlaveByteOrder=BigEndian  Direction=Receiver  RegisterAddressMode=on  RegisterAddress=MD25.MODE  SlaveDataType=uint8  DataLength=uint8(1)  NoAck=off  RepeatedStart=off  OutputStatus=off  SampleTime=SAMPLING_TIME
  Relational Operator : RelationalOperator  Operator===  OutDataTypeStr=boolean  RndMeth=Simplest  InputSameDT=off
  wires:
  MD25.MODE/1 -> Compare To Zero/1
  Constant3/1 -> MD25.MODE/1
  MD25.COMMAND 1/1 -> Compare To Zero1/1
  Constant6/1 -> MD25.COMMAND 1/1
  MD25.COMMAND 2/1 -> Compare To Zero2/1
  Constant9/1 -> MD25.COMMAND 2/1
  Compare To Zero/1 -> Logical Operator/1
  Compare To Zero1/1 -> Logical Operator/2
  Compare To Zero2/1 -> Logical Operator/3
  Constant10/1 -> MD25.COMMAND 3/1
  MD25.COMMAND 3/1 -> Compare To Zero3/1
  Compare To Zero3/1 -> Logical Operator/4
  Logical Operator/1 -> Data Store Write2/1
  MD25.MODE READ/1 -> Relational Operator/1
  Constant1/1 -> Relational Operator/2
  Relational Operator/1 -> Logical Operator/6
  MD25.ACCEL_RATE/1 -> Compare To Zero4/1
  Constant2/1 -> MD25.ACCEL_RATE/1
  Compare To Zero4/1 -> Logical Operator/5

== system CAR_CONTROL_SYSTEM/HARDWARE/ACTUATORS/MD25_I2C/READ BATTERY VOLTAGE ==
  Enable : EnablePort
  BATTERY VOLTAGE FILTER : MATLAB Function  Priority=30  TreatAsAtomicUnit=on
  Constant1 : Constant  Value=MD25.THR_NLFILT  VectorParams1D=off  OutDataTypeStr=double  SampleTime=SAMPLING_TIME
  Constant2 : Constant  Value=MD25.ALFA_FILT  VectorParams1D=off  OutDataTypeStr=double  SampleTime=SAMPLING_TIME
  Constant3 : Constant  Value=MD25.BATTERY_VOLT  VectorParams1D=off  OutDataTypeStr=double  SampleTime=SAMPLING_TIME
  Data Store Read : DataStoreRead  DataStoreName=CONTROL  SampleTime=SAMPLING_TIME  IndexOptions=Index vector (dialog)  Indices=1  OutputSizes=1
  Data Store Write : DataStoreWrite  DataStoreName=CONTROL  IndexOptions=Index vector (dialog)  Indices=1  OutputSizes=1
  Data Type Conversion1 : DataTypeConversion  OutDataTypeStr=double  SaturateOnIntegerOverflow=off  RndMeth=Floor
  Gain : Gain  Gain=0.1
  MD25.BATTERY_VOLTS : raspberrypiCommlib/I2C Controller Read  Priority=10  BoardProperty=Pi 3 Model B+  I2CModule=1  Mode=Master  SlaveAddress=MD25.ADDRESS  SlaveByteOrder=BigEndian  Direction=Receiver  RegisterAddressMode=on  RegisterAddress=MD25.BATTERY_VOLTS  SlaveDataType=uint8  DataLength=uint8(1)  NoAck=off  RepeatedStart=off  OutputStatus=off  SampleTime=SAMPLING_TIME
  wires:
  Data Store Read/1 -> BATTERY VOLTAGE FILTER/1(CONTROL_IN)
  BATTERY VOLTAGE FILTER/1(CONTROL) -> Data Store Write/1
  MD25.BATTERY_VOLTS/1 -> Data Type Conversion1/1
  Data Type Conversion1/1 -> Gain/1
  Gain/1 -> BATTERY VOLTAGE FILTER/2(BATTERY_VOLT)
  Constant3/1 -> BATTERY VOLTAGE FILTER/3(RATED_BATTERY_VOLT)
  Constant1/1 -> BATTERY VOLTAGE FILTER/4(THR_NLFILT)
  Constant2/1 -> BATTERY VOLTAGE FILTER/5(ALFA_FILT)

== system CAR_CONTROL_SYSTEM/HARDWARE/ACTUATORS/MD25_I2C/READ MOTOR CURRENT ==
  Enable : EnablePort
  Bus Assignment : BusAssignment  AssignedSignals=INPUT.MOTOR_CURRENT
  Data Store Read : DataStoreRead  DataStoreName=CONTROL  SampleTime=SAMPLING_TIME  IndexOptions=Index vector (dialog)  Indices=1  OutputSizes=1
  Data Store Write : DataStoreWrite  DataStoreName=CONTROL  IndexOptions=Index vector (dialog)  Indices=1  OutputSizes=1
  Data Type Conversion1 : DataTypeConversion  OutDataTypeStr=double  SaturateOnIntegerOverflow=off  RndMeth=Floor
  Gain : Gain  Gain=0.1
  MD25.MOTOR1_CURRENT : raspberrypiCommlib/I2C Controller Read  Priority=10  BoardProperty=Pi 3 Model B+  I2CModule=1  Mode=Master  SlaveAddress=MD25.ADDRESS  SlaveByteOrder=BigEndian  Direction=Receiver  RegisterAddressMode=on  RegisterAddress=MD25.MOTOR1_CURRENT  SlaveDataType=uint8  DataLength=uint8(2)  NoAck=off  RepeatedStart=off  OutputStatus=off  SampleTime=SAMPLING_TIME
  wires:
  Data Store Read/1 -> Bus Assignment/1
  Bus Assignment/1 -> Data Store Write/1
  Data Type Conversion1/1 -> Gain/1
  Gain/1 -> Bus Assignment/2
  MD25.MOTOR1_CURRENT/1 -> Data Type Conversion1/1

== system CAR_CONTROL_SYSTEM/HARDWARE/ACTUATORS/MD25_I2C/READ MOTOR ENCODER ==
  Enable : EnablePort
  Data Store Read : DataStoreRead  DataStoreName=CONTROL  SampleTime=SAMPLING_TIME  IndexOptions=Index vector (dialog)  Indices=1  OutputSizes=1
  Data Store Write1 : DataStoreWrite  DataStoreName=CONTROL  IndexOptions=Index vector (dialog)  Indices=1  OutputSizes=1
  MD25.ENC1A : raspberrypiCommlib/I2C Controller Read  Priority=10  BoardProperty=Pi 3 Model B+  I2CModule=1  Mode=Master  SlaveAddress=MD25.ADDRESS  SlaveByteOrder=BigEndian  Direction=Receiver  RegisterAddressMode=on  RegisterAddress=MD25.ENC1A  SlaveDataType=uint8  DataLength=uint8(8)  NoAck=off  RepeatedStart=off  OutputStatus=off  SampleTime=SAMPLING_TIME
  READ ENCODER ANGLE : MATLAB Function  Commented=on  TreatAsAtomicUnit=on
  READ_ENCODER : MATLAB Function  TreatAsAtomicUnit=on
  READ_ENCODER OLD : MATLAB Function  Commented=on  TreatAsAtomicUnit=on
  wires:
  Data Store Read/1 -> READ_ENCODER/1(CONTROL_IN)
  READ_ENCODER/1(CONTROL) -> Data Store Write1/1
  MD25.ENC1A/1 -> READ_ENCODER/2(MOTOR_ENC_BYTES)

== system CAR_CONTROL_SYSTEM/HARDWARE/ACTUATORS/MD25_I2C/RESET MOTOR ENCODER ==
  Enable : EnablePort
  Constant6 : Constant  Value=hex2dec('20')  OutDataTypeStr=uint8  SampleTime=SAMPLING_TIME
  MD25.COMMAND 1 : raspberrypiCommlib/I2C Controller Write  BoardProperty=Pi 3 Model B+  I2CModule=1  Mode=Master  SlaveAddress=MD25.ADDRESS  SlaveByteOrder=BigEndian  Direction=Transmitter  RegisterAddressMode=on  RegisterAddress=MD25.COMMAND  SlaveDataType=uint8  DataLength=1  NoAck=off  RepeatedStart=off  OutputStatus=off
  wires:
  Constant6/1 -> MD25.COMMAND 1/1

== system CAR_CONTROL_SYSTEM/HARDWARE/ACTUATORS/MD25_I2C/WRITE PWM MOTOR  ==
  Enable : EnablePort
  Bus Assignment : BusAssignment  AssignedSignals=OUTPUT.MOTOR_PWM
  Constant2 : Constant  Commented=on  Value=hex2dec('10')  OutDataTypeStr=uint8  SampleTime=SAMPLING_TIME
  Constant5 : Constant  Value=MD25.PWM_MAX  OutDataTypeStr=double  SampleTime=SAMPLING_TIME
  Constant6 : Constant  Value=MD25.PWM_MIN  OutDataTypeStr=double  SampleTime=SAMPLING_TIME
  Data Store Read1 : DataStoreRead  DataStoreName=CONTROL  SampleTime=SAMPLING_TIME  IndexOptions=Index vector (dialog)  Indices=1  OutputSizes=1
  Data Store Read2 : DataStoreRead  DataStoreName=CONTROL  SampleTime=SAMPLING_TIME  IndexOptions=Index vector (dialog)  Indices=1  OutputSizes=1
  Data Store Write1 : DataStoreWrite  DataStoreName=CONTROL  IndexOptions=Index vector (dialog)  Indices=1  OutputSizes=1
  Demux : Demux  Outputs=2
  MD25.ACCEL_RATE : raspberrypiCommlib/I2C Controller Write  Priority=0  Commented=on  BoardProperty=Pi 3 Model B+  I2CModule=1  Mode=Master  SlaveAddress=MD25.ADDRESS  SlaveByteOrder=BigEndian  Direction=Transmitter  RegisterAddressMode=on  RegisterAddress=MD25.ACCEL_RATE  SlaveDataType=uint8  DataLength=1  NoAck=off  RepeatedStart=off  OutputStatus=off
  MD25.SPEED1 : raspberrypiCommlib/I2C Controller Write  BoardProperty=Pi 3 Model B+  I2CModule=1  Mode=Master  SlaveAddress=MD25.ADDRESS  SlaveByteOrder=BigEndian  Direction=Transmitter  RegisterAddressMode=on  RegisterAddress=MD25.SPEED1  SlaveDataType=uint8  DataLength=1  NoAck=off  RepeatedStart=off  OutputStatus=off
  MD25.SPEED2 : raspberrypiCommlib/I2C Controller Write  BoardProperty=Pi 3 Model B+  I2CModule=1  Mode=Master  SlaveAddress=MD25.ADDRESS  SlaveByteOrder=BigEndian  Direction=Transmitter  RegisterAddressMode=on  RegisterAddress=MD25.SPEED2  SlaveDataType=uint8  DataLength=1  NoAck=off  RepeatedStart=off  OutputStatus=off
  PWM CONVERSION : MATLAB Function  TreatAsAtomicUnit=on
  wires:
  Constant5/1 -> PWM CONVERSION/2(PWM_MAX)
  Constant6/1 -> PWM CONVERSION/3(PWM_MIN)
  PWM CONVERSION/1(PWM_BYTE) -> Demux/1
  Data Store Read1/1 -> Bus Assignment/1
  Bus Assignment/1 -> Data Store Write1/1
  PWM CONVERSION/2(MOTOR_PWM) -> Bus Assignment/2
  Demux/2 -> MD25.SPEED1/1
  Demux/1 -> MD25.SPEED2/1
  Constant2/1 -> MD25.ACCEL_RATE/1
  Data Store Read2/1 -> PWM CONVERSION/1(CONTROL)

== system CAR_CONTROL_SYSTEM/HARDWARE/COMMUNICATIONS/TCP//IP/MSG_RX ==
  Bus Assignment : BusAssignment  AssignedSignals=RX_BUFFER
  Data Store Read : DataStoreRead  DataStoreName=MSG  IndexOptions=Index vector (dialog)  Indices=1  OutputSizes=1
  Data Store Write1 : DataStoreWrite  DataStoreName=MSG  IndexOptions=Index vector (dialog)  Indices=1  OutputSizes=1
  TCP/IP Receive : raspberrypiNetworklib/TCP//IP Receive  Mode_=Server  LocalServerPort_=27001  RemoteAddr_=127.0.0.1  RemoteServerPort_=25000  DataType_=uint8  DataSize_=1400  SampleTime_=CONTROL_INI.PARAM.COMM_SAMPLING_TIME  SimulateUsing=Code generation  ClientPortBindingSelection_=off  ClientPortToBind_=35000  BlockingMode_=off  BlockTimeout_=0.1  BlockPlatform=RASPBERRYPI
  Terminator1 : Terminator
  wires:
  TCP/IP Receive/1 -> Bus Assignment/2
  Data Store Read/1 -> Bus Assignment/1
  Bus Assignment/1 -> Data Store Write1/1
  TCP/IP Receive/2 -> Terminator1/1

== system CAR_CONTROL_SYSTEM/HARDWARE/COMMUNICATIONS/TCP//IP/MSG_TX ==
  Enable : EnablePort
  Data Store Read1 : DataStoreRead  DataStoreName=MSG  SampleTime=CONTROL_INI.PARAM.COMM_SAMPLING_TIME  DataStoreElements=MSG.TX_BUFFER(:,1)  IndexOptions=Index vector (dialog)  Indices=1  OutputSizes=1
  TCP/IP Send : raspberrypiNetworklib/TCP//IP Send  Mode_=Server  LocalServerPort_=27000  RemoteAddr_=127.0.0.1  RemoteServerPort_=25000  SimulateUsing=Code generation  ClientPortBindingSelection_=off  ClientPortToBind_=35000  BlockingMode_=off  BlockTimeout_=0.1  BlockPlatform=RASPBERRYPI
  wires:
  Data Store Read1/1 -> TCP/IP Send/1

== system CAR_CONTROL_SYSTEM/HARDWARE/SENSORS/IMU MPU60X0_SPI/INITIALIZATION ==
  Enable : EnablePort
  Compare To Constant : simulink/Logic and Bit Operations/Compare To Constant  relop===  const=MPU60X0.CONFIG_BYTE  OutDataTypeStr=boolean
  Data Store Write : DataStoreWrite  DataStoreName=MPU60X0_INIT  IndexOptions=Index vector (dialog)  Indices=1  OutputSizes=1
  MPU9250.ACCEL_CONFIG : raspberrypiCommlib/SPI Register Write  Priority=50  BoardProperty=Pi 3 Model B+  SSPin=SPI0_CE1  SPIModule=uint32(0)  Mode=Master  BusSpeed=1000000  Pin=SPI0_CE0  FirstBitToTransfer=Most significant bit (MSB)  ClockMode=3  BlockFunction=Write  RegisterAddress=MPU60X0.ACCEL_CONFIG  OutputDataType=int8  OutputDataLength=1
  MPU9250.CONFIG : raspberrypiCommlib/SPI Register Write  Priority=80  BoardProperty=Pi 3 Model B+  SSPin=SPI0_CE1  SPIModule=uint32(0)  Mode=Master  BusSpeed=1000000  Pin=SPI0_CE0  FirstBitToTransfer=Most significant bit (MSB)  ClockMode=3  BlockFunction=Write  RegisterAddress=MPU60X0.CONFIG  OutputDataType=int8  OutputDataLength=1
  MPU9250.FIFO_EN : raspberrypiCommlib/SPI Register Write  Priority=70  BoardProperty=Pi 3 Model B+  SSPin=SPI0_CE1  SPIModule=uint32(0)  Mode=Master  BusSpeed=1000000  Pin=SPI0_CE0  FirstBitToTransfer=Most significant bit (MSB)  ClockMode=3  BlockFunction=Write  RegisterAddress=MPU60X0.FIFO_EN  OutputDataType=int8  OutputDataLength=1
  MPU9250.GYRO_CONFIG : raspberrypiCommlib/SPI Register Write  Priority=60  BoardProperty=Pi 3 Model B+  SSPin=SPI0_CE1  SPIModule=uint32(0)  Mode=Master  BusSpeed=1000000  Pin=SPI0_CE0  FirstBitToTransfer=Most significant bit (MSB)  ClockMode=3  BlockFunction=Write  RegisterAddress=MPU60X0.GYRO_CONFIG  OutputDataType=int8  OutputDataLength=1
  MPU9250.INT_ENABLE : raspberrypiCommlib/SPI Register Write  Priority=40  BoardProperty=Pi 3 Model B+  SSPin=SPI0_CE1  SPIModule=uint32(0)  Mode=Master  BusSpeed=1000000  Pin=SPI0_CE0  FirstBitToTransfer=Most significant bit (MSB)  ClockMode=3  BlockFunction=Write  RegisterAddress=MPU60X0.INT_ENABLE  OutputDataType=int8  OutputDataLength=1
  MPU9250.PWR_MGMT_1 : raspberrypiCommlib/SPI Register Write  Priority=20  BoardProperty=Pi 3 Model B+  SSPin=SPI0_CE1  SPIModule=uint32(0)  Mode=Master  BusSpeed=1000000  Pin=SPI0_CE0  FirstBitToTransfer=Most significant bit (MSB)  ClockMode=3  BlockFunction=Write  RegisterAddress=MPU60X0.PWR_MGMT_1  OutputDataType=int8  OutputDataLength=1
  MPU9250.SMPLRT_DIV : raspberrypiCommlib/SPI Register Write  Priority=30  BoardProperty=Pi 3 Model B+  SSPin=SPI0_CE1  SPIModule=uint32(0)  Mode=Master  BusSpeed=1000000  Pin=SPI0_CE0  FirstBitToTransfer=Most significant bit (MSB)  ClockMode=3  BlockFunction=Write  RegisterAddress=MPU60X0.SMPLRT_DIV  OutputDataType=int8  OutputDataLength=1
  MPU9250.USER_CTRL : raspberrypiCommlib/SPI Register Write  Priority=10  BoardProperty=Pi 3 Model B+  SSPin=SPI0_CE1  SPIModule=uint32(0)  Mode=Master  BusSpeed=1000000  Pin=SPI0_CE0  FirstBitToTransfer=Most significant bit (MSB)  ClockMode=3  BlockFunction=Write  RegisterAddress=MPU60X0.USER_CTRL  OutputDataType=int8  OutputDataLength=1
  OUT_X_L1 : Constant  Value=MPU60X0.CONFIG_BYTE  OutDataTypeStr=uint8  SampleTime=-1
  OUT_X_L2 : Constant  Value=MPU60X0.INT_ENABLE_BYTE  OutDataTypeStr=uint8  SampleTime=-1
  OUT_X_L21 : Constant  Value=MPU60X0.FIFO_EN_BYTE  OutDataTypeStr=uint8  SampleTime=-1
  OUT_X_L22 : Constant  Value=MPU60X0.USER_CTRL_BYTE  OutDataTypeStr=uint8  SampleTime=-1
  OUT_X_L23 : Constant  Value=MPU60X0.PWR_MGMT_1_BYTE  OutDataTypeStr=uint8  SampleTime=-1
  OUT_X_L24 : Constant  Value=MPU60X0.SMPLRT_DIV_BYTE  OutDataTypeStr=uint8  SampleTime=-1
  OUT_X_L8 : Constant  Value=MPU60X0.ACCEL_CONFIG_BYTE  OutDataTypeStr=uint8  SampleTime=-1
  OUT_X_L9 : Constant  Value=MPU60X0.GYRO_CONFIG_BYTE  OutDataTypeStr=uint8  SampleTime=-1
  Subsystem : Subsystem  Priority=90  mask{Register=MPU60X0.CONFIG, n=1}
      mask prompts: Register "MPU9250 Register"; n "Data size (bytes)"
  wires:
  Compare To Constant/1 -> Data Store Write/1
  Subsystem/1(Out1) -> Compare To Constant/1
  OUT_X_L8/1 -> MPU9250.ACCEL_CONFIG/1
  OUT_X_L23/1 -> MPU9250.PWR_MGMT_1/1
  OUT_X_L21/1 -> MPU9250.FIFO_EN/1
  OUT_X_L22/1 -> MPU9250.USER_CTRL/1
  OUT_X_L2/1 -> MPU9250.INT_ENABLE/1
  OUT_X_L9/1 -> MPU9250.GYRO_CONFIG/1
  OUT_X_L24/1 -> MPU9250.SMPLRT_DIV/1
  OUT_X_L1/1 -> MPU9250.CONFIG/1

== system CAR_CONTROL_SYSTEM/HARDWARE/SENSORS/IMU MPU60X0_SPI/READ FIFO ==
  Enable : EnablePort
  Constant2 : Constant  Commented=on  Value=bin2dec('01000100');  OutDataTypeStr=uint8  SampleTime=SAMPLING_TIME
  Constant3 : Constant  Value=MPU60X0.ACCEL_SSF  SampleTime=SAMPLING_TIME
  Constant4 : Constant  Value=MPU60X0.GYRO_SSF  SampleTime=SAMPLING_TIME
  Constant7 : Constant  Value=MPU60X0.FIFO_LENGTH  OutDataTypeStr=uint8  SampleTime=SAMPLING_TIME
  Data Store Read : DataStoreRead  DataStoreName=CONTROL  DataStoreElements=CONTROL_BUS.INPUT.IMU.ACCEL_MEAN(:,:)#CONTROL_BUS.INPUT.IMU.GYRO_MEAN(:,:)  IndexOptions=Index vector (dialog)  Indices=1  OutputSizes=1
  Data Store Read2 : DataStoreRead  DataStoreName=CONTROL  SampleTime=SAMPLING_TIME  IndexOptions=Index vector (dialog)  Indices=1  OutputSizes=1
  Data Store Write : DataStoreWrite  DataStoreName=CONTROL  IndexOptions=Index vector (dialog)  Indices=1  OutputSizes=1
  Data Store Write1 : DataStoreWrite  DataStoreName=MPU60X0_RAW_GYRO_MEAN  IndexOptions=Index vector (dialog)  Indices=1  OutputSizes=1
  Data Store Write2 : DataStoreWrite  DataStoreName=MPU60X0_RAW_ACCEL_MEAN  IndexOptions=Index vector (dialog)  Indices=1  OutputSizes=1
  Data Type Conversion : DataTypeConversion  OutDataTypeStr=double  SaturateOnIntegerOverflow=off  RndMeth=Floor
  Data Type Conversion4 : DataTypeConversion  OutDataTypeStr=int16  SaturateOnIntegerOverflow=off  RndMeth=Floor
  EVEN POSITIONS : Selector  InputPortWidth=uint8(12*MPU9250.FIFO_LENGTH)  IndexOptions=Index vector (dialog)  Indices=2:2:uint8(12*MPU9250.FIFO_LENGTH)  OutputSizes=1
  FIFO READ : Subsystem  mask{Register=MPU60X0.FIFO_R_W, n=12*MPU60X0.FIFO_LENGTH}
      mask prompts: Register "MPU9250 Register"; n "Data size (bytes)"
      mask DialogControl Control2 Prompt: (Add text here)
  FIFO RESET : raspberrypiCommlib/SPI Register Write  Priority=20  Commented=on  BoardProperty=Pi 3 Model B+  SSPin=SPI0_CE1  SPIModule=uint32(0)  Mode=Master  BusSpeed=1000000  Pin=SPI0_CE0  FirstBitToTransfer=Most significant bit (MSB)  ClockMode=3  BlockFunction=Write  RegisterAddress=MPU60X0.USER_CTRL  OutputDataType=int8  OutputDataLength=1
  FIFO_PROCESSING : MATLAB Function  Priority=30  TreatAsAtomicUnit=on
  Gain61 : Gain  Gain=2^8
  Mux : Mux
  ODD POSITIONS : Selector  InputPortWidth=uint8(12*MPU9250.FIFO_LENGTH)  IndexOptions=Index vector (dialog)  Indices=1:2:uint8(12*MPU9250.FIFO_LENGTH)  OutputSizes=1
  Sum61 : Sum  Inputs=|++
  To File : ToFile  Filename=BLACK_BOX_FIFO.mat  MatrixName=FIFO_LOG
  wires:
  Data Store Read/2 -> Mux/4
  Data Store Read/1 -> Mux/3
  FIFO_PROCESSING/5(GYRO_FIFO) -> Mux/2
  FIFO_PROCESSING/4(ACCEL_FIFO) -> Mux/1
  Constant4/1 -> FIFO_PROCESSING/5(GYRO_SSF)
  Constant3/1 -> FIFO_PROCESSING/4(ACCEL_SSF)
  Mux/1 -> Data Type Conversion/1
  Data Type Conversion/1 -> To File/1
  Data Type Conversion4/1 -> FIFO_PROCESSING/2(FIFO_DATA)
  FIFO READ/1(Out1) -> ODD POSITIONS/1, EVEN POSITIONS/1
  FIFO_PROCESSING/3(RAW_ACCEL_MEAN_OUT) -> Data Store Write2/1
  FIFO_PROCESSING/2(RAW_GYRO_MEAN_OUT) -> Data Store Write1/1
  Constant2/1 -> FIFO RESET/1
  Data Store Read2/1 -> FIFO_PROCESSING/1(CONTROL_IN)
  Sum61/1 -> Data Type Conversion4/1
  FIFO_PROCESSING/1(CONTROL_OUT) -> Data Store Write/1
  Constant7/1 -> FIFO_PROCESSING/3(FIFO_LENGTH)
  EVEN POSITIONS/1 -> Sum61/2
  Gain61/1 -> Sum61/1
  ODD POSITIONS/1 -> Gain61/1
